simulink model "sl_groundvehicleDynamics"  (R2025a)
settings: Solver=ode45  StartTime=0.0  StopTime=2000  RelTol=1e-5  EnableMultiTasking=on
InitFcn:
  | mdl_robot;
values from neighbouring files (symbols this model uses):
  Ordered_Waypoints = cell2mat({WP_List.Pos}')    [Waypoint_Generator.m]
undefined symbols (not defined in the file or in its folder): DiscIntNeverNeededParam, robot
libraries: simulink x4, mobileRoboticsLib x3, simulink_extras x2
settings Model: Creator=sriramn  LastModifiedBy=Education Account
settings SolverCC: ZeroCrossAlgorithm=Adaptive  AlgebraicLoopSolver=TrustRegion
settings DataIOCC: LimitDataPoints=on  SaveFormat=Array  ReturnWorkspaceOutputs=off
settings OptimizationCC: ReuseModelBlockBuffer=off  LifeSpan=inf
settings DebuggingCC: SolverPrmCheckMsg=warning  UnconnectedInputMsg=warning  UnconnectedOutputMsg=warning  UnconnectedLineMsg=warning  AllowSymbolicDim=off  SFUnexpectedBacktrackingDiag=warning  SFNoUnconditionalDefaultTransitionDiag=warning  SFExecutionAtInitializationDiag=none  UnderSpecifiedDimensionMsg=warning  ArithmeticOperatorsInVariantConditions=warning
settings HardwareCC: ProdBitPerPointer=32.0  ProdBitPerSizeT=32.0  ProdBitPerPtrDiffT=32.0  ProdLargestAtomicFloat=None  ProdIntDivRoundTo=Undefined  ProdEndianess=Unspecified  ProdWordSize=32.0  ProdHWDeviceType=32-bit Generic
settings ModelReferenceCC: EnableRefExpFcnMdlSchedulingChecks=on  ModelReferenceMinAlgLoopOccurrences=on  PropagateSignalLabelsOutOfModel=off
settings SFSimCC: SimUseLocalCustomCode=off  CustomCodeUndefinedFunction=UseInterfaceOnly
settings RTWCC: RTWUseLocalCustomCode=off  GPUComputeCapability=3.5
settings CodeAppCC: StateflowObjectComments=on
settings GRTTargetCC: TargetLangStandard=C89/C90 (ANSI)
settings ConfigComp: CovMetricSettings=dw  CovSaveCumulativeToWorkspaceVar=on  CovSaveSingleToWorkspaceVar=on  CovExternalEMLEnable=off  CovSFcnEnable=off
settings SimscapeCC: SimscapeNormalizeSystem=off
settings ConfigurationSet: Description=SimMechanics 2G
settings ExplorerConfigSet: InternalSimMechanicsExplorerSettings="<ExplorerConfiguration><canonicalview>planar_xy</canonicalview><AnimationSetting><BasePlaybackSpeed>1.0</BasePlaybackSpeed><PlaybackSpeedFactor>1.0</PlaybackSpeedFactor></AnimationSetting><TilePanel><TileInfo><Tiles Columns=\"1\" Count=\"1\" Rows=\"1\"><Column Left=\"2\" Weight=\"1\"/><Column Left=\"1628\"/><Row Top=\"2\" Weight=\"1\"/><Row Top=\"1072\"/><Tile Height=\"1\" Width=\"1\" X=\"0\" Y=\"0\"/></Tiles></TileInfo><SceneInfo><SceneViewer><BGColor><R>0.60000002384185791</R><G>0.60000002384185791</G><B>0.60000002384185791</B></BGColor><Camera><Position><X>0.22951840878551699</X><Y>0.32651610611526627</Y><Z>-0.27215421354393321</Z></Position><Center><X>-0.15775714411666431</X><Y>-0.15462825985839526</Y><Z>0.065702552916005602</Z></Center><Up><X>-0.56030137557930915</X><Y>0.72817587161684794</Y><Z>0.39474329445726858</Z></Up><Left>-0.21481383955700509</Left><Right>0.21481383955700509</Right><Bottom>-0.27569784609469139</Bottom><Top>0.27569784609469139</Top></Camera></SceneViewer></SceneInfo></TilePanel></ExplorerConfiguration>"

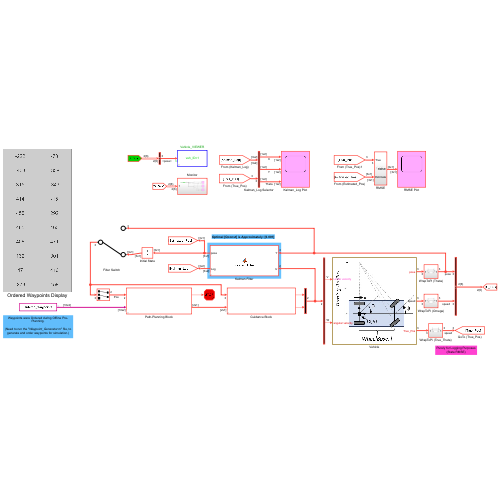
[thumbnail: Simulink's stored preview of the top-level diagram]
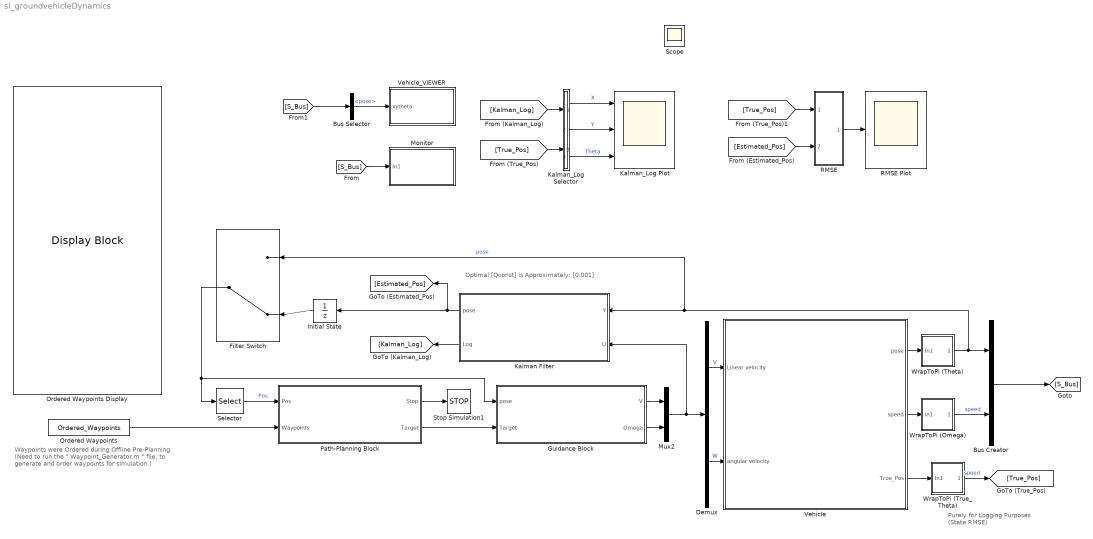
== system sl_groundvehicleDynamics ==
  note: Optimal [Qconst] is Approximately: [0.001]
  note: Waypoints were Ordered during Offline Pre-Planning.
      |
      | (Need to run the " Waypoint_Generator.m " file, to generate and order waypoints for simulation.)
  note: Purely for Logging Purposes
      | (State RMSE)
  Bus Creator : BusCreator  Inputs=2
  Bus Selector : BusSelector  OutputSignals=pose
  Demux : Demux  Outputs=2
  Filter Switch : ManualSwitch  CurrentSetting=0
  Guidance Block : MATLAB Function  TreatAsAtomicUnit=on  mask{Vc=10, MaxOmega=90, Kp=10, Kd=0, N=4, dT=0.05}
      mask prompts: Vc "Linear Velocity (m/s):"; MaxOmega "Maximum Angular Velocity (deg/s):"; Kp "Proportional Gain [Kp]:"; Kd "Derivative Gain [Kd] (ignore):"; N "Navigation Gain [N] (ignore):"; dT "Sample Time [dT]:"
  Initial State : UnitDelay  InitialCondition=[0; 0; 0]  SampleTime=0.05  HasFrameUpgradeWarning=on
  Kalman Filter : MATLAB Function  TreatAsAtomicUnit=on  SystemSampleTime=0.05  mask{sig2_V=10^-3, sig2_W=10^-3, P0_pos=100, P0_theta=100, dT=0.05}
      mask prompts: sig2_V "Linear Velocity Variance [sig2_V]:"; sig2_W "Angular Velocity Variance [sig2_W]:"; P0_pos "Initial Position Variance [P0_pos]:"; P0_theta "Initial Heading Variance [P0_theta]:"; dT "Sample Time [dT]:"
  Kalman_Log Plot : Scope  NumInputPorts=3
      settings: SampleTime=0.05  TimeSpan=350  ActiveDisplayYMinimum=-0.45488119893113321  ActiveDisplayYMaximum=0.48875254754884168
  Kalman_Log Selector : Subsystem
  Monitor : Subsystem
  Mux2 : Mux  Inputs=2
  Ordered Waypoints : Constant  Value=Ordered_Waypoints  VectorParams1D=off
  Ordered Waypoints Display : DisplayBlock  LabelPosition=Hide  Transparency=1  GridColor=[0.502, 0.502, 0.502]
  Path-Planning Block : MATLAB Function  TreatAsAtomicUnit=on  mask{LookAhead=5, WP_Thresh=20}
      mask prompts: LookAhead "Look-Ahead Distance [Ahead]:"; WP_Thresh "WayPoint Threshold [WP_Thresh]:"
  RMSE : Subsystem
  RMSE Plot : Scope
      settings: SampleTime=0.05  TimeSpan=700  Title=State Estimation RMSE  ActiveDisplayYMinimum=-0.13363764478764484  ActiveDisplayYMaximum=1.9663623552123544  YLabel=RMSE  DataLoggingVariableName=ScopeData3
  Selector : Selector  InputPortWidth=3  IndexOptions=Index vector (dialog)  Indices=[1 2]  OutputSizes=1
  Stop Simulation1 : Stop
  Vehicle : Subsystem
      mask Display: image('vehicle.jpg');
  Vehicle_VIEWER : Subsystem  mask{wp_mat=[-500, 500; -500, 500]', veh_ID_num=1, veh_init_xytheta=[robot.X robot.Y robot.Theta], Ts=0.5}
      mask prompts: wp_mat "Waypoint matrix for arena [x_col, y_col] (m)"; veh_ID_num "Vehicle ID number"; veh_init_xytheta "Initial pose [x,y,theta]"; Ts "Sample time for updating animation (secs)"
      mask TypeOptions veh_ID_num: 1 | 2 | 3 | 4
      mask DialogControl Control2 Prompt: Animate simulation of Differential Drive Robot (DDR)
      mask Display: fprintf('veh_ID=%d',veh_ID_num);
  WrapToPi (Omega) : Subsystem
  WrapToPi (Theta) : Subsystem
  WrapToPi (True_Theta) : Subsystem
  Scope : Scope
      settings: ActiveDisplayYMinimum=0.07  ActiveDisplayYMaximum=0.09
  wires:
  [S_Bus] -> Monitor/1(In1)
  [S_Bus] -> Bus Selector/1
  Vehicle/2(speed) -> WrapToPi (Omega)/1(In1)
  Bus Creator/1 -> [S_Bus]
  Bus Selector/1 -> Vehicle_VIEWER/1(xytheta)  "<pose>"
  Demux/1 -> Vehicle/1(Linear velocity)  "V"
  Guidance Block/2(Omega) -> Mux2/2
  Guidance Block/1(V) -> Mux2/1
  Demux/2 -> Vehicle/2(angular velocity)  "W"
  Mux2/1 -> Kalman Filter/2(U), Demux/1
  Path-Planning Block/2(Target) -> Guidance Block/2(Target)
  Ordered Waypoints/1 -> Path-Planning Block/2(Waypoints)
  Vehicle/1(pose) -> WrapToPi (Theta)/1(In1)
  Path-Planning Block/1(Stop) -> Stop Simulation1/1
  Kalman Filter/1(pose) -> [Estimated_Pos], Initial State/1
  Filter Switch/1 -> Guidance Block/1(pose), Selector/1
  Selector/1 -> Path-Planning Block/1(Pos)  "Pos"
  Kalman_Log Selector/2(Y) -> Kalman_Log Plot/2  "Y"
  Kalman_Log Selector/1(X) -> Kalman_Log Plot/1  "X"
  Kalman_Log Selector/3(Theta) -> Kalman_Log Plot/3  "Theta"
  [Kalman_Log] -> Kalman_Log Selector/1(Log)
  WrapToPi (Theta)/1(Out1) -> Bus Creator/1, Kalman Filter/1(Y), Filter Switch/1  "pose"
  WrapToPi (Omega)/1(Out1) -> Bus Creator/2  "speed"
  Initial State/1 -> Filter Switch/2
  Kalman Filter/2(Log) -> [Kalman_Log]
  Vehicle/3(True_Pos) -> WrapToPi (True_Theta)/1(In1)
  [True_Pos] -> Kalman_Log Selector/2(True_Pos)
  WrapToPi (True_Theta)/1(Out1) -> [True_Pos]  "speed"
  [True_Pos] -> RMSE/1(True)
  [Estimated_Pos] -> RMSE/2(Estimate)
  RMSE/1(RMSE) -> RMSE Plot/1

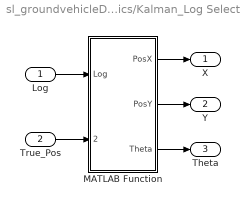
== system sl_groundvehicleDynamics/Kalman_Log Selector ==
  Log : Inport
  True_Pos : Inport  Port=2
  MATLAB Function : MATLAB Function  TreatAsAtomicUnit=on
  X : Outport
  Y : Outport  Port=2
  Theta : Outport  Port=3
  wires:
  MATLAB Function/1(PosX) -> X/1
  MATLAB Function/2(PosY) -> Y/1
  MATLAB Function/3(Theta) -> Theta/1
  Log/1 -> MATLAB Function/1(Log)
  True_Pos/1 -> MATLAB Function/2(True_Pos)

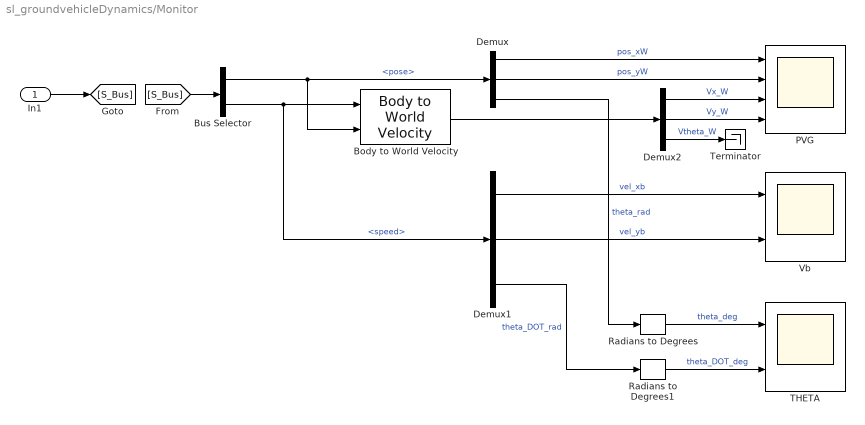
== system sl_groundvehicleDynamics/Monitor ==
  In1 : Inport
  Body to World Velocity : mobileRoboticsLib/Utilities/Body to World Velocity
      settings: SourceProductName=Mobile Robotics Simulation Toolbox
  Bus Selector : BusSelector  OutputSignals=pose,speed
  Demux : Demux  Outputs=3
  Demux1 : Demux  Outputs=3
  Demux2 : Demux  Outputs=3
  PVG : Scope  NumInputPorts=4
      settings: ActiveDisplayYMinimum=-5.1706239874781605  ActiveDisplayYMaximum=31.754450302209349
  Radians to Degrees : simulink_extras/Transformations/Radians to Degrees
  Radians to Degrees1 : simulink_extras/Transformations/Radians to Degrees
  THETA : Scope  NumInputPorts=2
      settings: ActiveDisplayYMinimum=-8.72937  ActiveDisplayYMaximum=60.06611  DataLoggingVariableName=ScopeData2
  Terminator : Terminator
  Vb : Scope  NumInputPorts=2
      settings: ActiveDisplayYMinimum=0.05577  ActiveDisplayYMaximum=0.8929
  wires:
  In1/1 -> [S_Bus]
  [S_Bus] -> Bus Selector/1
  Demux/1 -> PVG/1  "pos_xW"
  Demux/2 -> PVG/2  "pos_yW"
  Radians to Degrees1/1 -> THETA/2  "theta_DOT_deg"
  Radians to Degrees/1 -> THETA/1  "theta_deg"
  Demux1/3 -> Radians to Degrees1/1  "theta_DOT_rad"
  Demux/3 -> Radians to Degrees/1  "theta_rad"
  Bus Selector/1 -> Body to World Velocity/2, Demux/1  "<pose>"
  Bus Selector/2 -> Demux1/1, Body to World Velocity/1  "<speed>"
  Body to World Velocity/1 -> Demux2/1
  Demux2/1 -> PVG/3  "Vx_W"
  Demux2/2 -> PVG/4  "Vy_W"
  Demux1/1 -> Vb/1  "vel_xb"
  Demux1/2 -> Vb/2  "vel_yb"
  Demux2/3 -> Terminator/1  "Vtheta_W"

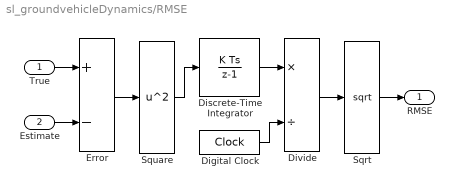
== system sl_groundvehicleDynamics/RMSE ==
  True : Inport
  Estimate : Inport  Port=2
  Digital Clock : DigitalClock  SampleTime=0.05
  Discrete-Time Integrator : DiscreteIntegrator  SampleTime=0.05  ICPrevOutput=DiscIntNeverNeededParam  ICPrevScaledInput=DiscIntNeverNeededParam
  Divide : Product  Inputs=*/
  Error : Sum  Inputs=+-
  Sqrt : Sqrt
  Square : Math  Operator=square
  RMSE : Outport
  wires:
  True/1 -> Error/1
  Estimate/1 -> Error/2
  Divide/1 -> Sqrt/1
  Digital Clock/1 -> Divide/2
  Square/1 -> Discrete-Time Integrator/1
  Error/1 -> Square/1
  Discrete-Time Integrator/1 -> Divide/1
  Sqrt/1 -> RMSE/1

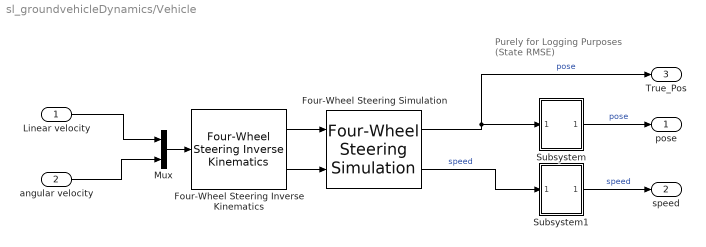
== system sl_groundvehicleDynamics/Vehicle ==
  note: Purely for Logging Purposes
      | (State RMSE)
  Linear velocity : Inport
  angular velocity : Inport  Port=2
  Four-Wheel Steering Inverse Kinematics : mobileRoboticsLib/Kinematic Models/Four-Wheel Steering/Four-Wheel Steering Inverse Kinematics  wheelRadius=0.1  frontWheelDist=0.25  rearWheelDist=0.25  ikMode=Front Steering
      settings: SourceProductName=Mobile Robotics Simulation Toolbox
  Four-Wheel Steering Simulation : mobileRoboticsLib/Kinematic Models/Four-Wheel Steering/Four-Wheel Steering Simulation  wheelRadius=0.1  frontWheelDist=0.25  rearWheelDist=0.25  initX=robot.X  initY=robot.Y  initAngle=robot.Theta  Ts=0.05
      settings: SourceProductName=Mobile Robotics Simulation Toolbox
  Mux : Mux  Inputs=2
  Subsystem : Subsystem
  Subsystem1 : Subsystem
  pose : Outport  VectorParamsAs1DForOutWhenUnconnected=off
  speed : Outport  Port=2
  True_Pos : Outport  Port=3  VectorParamsAs1DForOutWhenUnconnected=off
  wires:
  angular velocity/1 -> Mux/2
  Linear velocity/1 -> Mux/1
  Mux/1 -> Four-Wheel Steering Inverse Kinematics/1
  Four-Wheel Steering Simulation/1 -> True_Pos/1, Subsystem/1(In1)  "pose"
  Four-Wheel Steering Simulation/2 -> Subsystem1/1(In1)  "speed"
  Four-Wheel Steering Inverse Kinematics/1 -> Four-Wheel Steering Simulation/1
  Four-Wheel Steering Inverse Kinematics/2 -> Four-Wheel Steering Simulation/2
  Subsystem/1(pose) -> pose/1  "pose"
  Subsystem1/1(speed) -> speed/1  "speed"

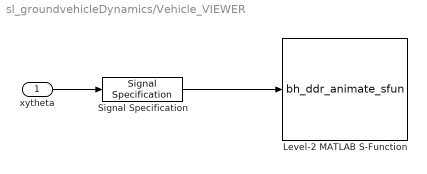
== system sl_groundvehicleDynamics/Vehicle_VIEWER ==
  xytheta : Inport
  Level-2 MATLAB S-Function : M-S-Function  FunctionName=bh_ddr_animate_sfun  Parameters=Ts, Ordered_Waypoints, veh_ID_num, veh_init_xytheta
  Signal Specification : SignalSpecification  Dimensions=3
  wires:
  xytheta/1 -> Signal Specification/1
  Signal Specification/1 -> Level-2 MATLAB S-Function/1

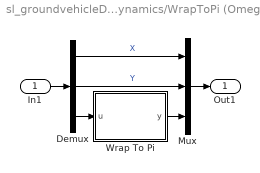
== system sl_groundvehicleDynamics/WrapToPi (Omega) ==
  In1 : Inport
  Demux : Demux  Outputs=3
  Mux : Mux  Inputs=3
  Wrap To Pi : MATLAB Function  TreatAsAtomicUnit=on
  Out1 : Outport
  wires:
  In1/1 -> Demux/1
  Mux/1 -> Out1/1
  Demux/1 -> Mux/1  "X"
  Demux/2 -> Mux/2  "Y"
  Demux/3 -> Wrap To Pi/1(u)
  Wrap To Pi/1(y) -> Mux/3

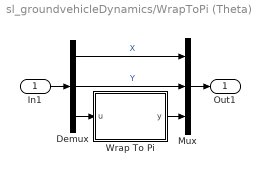
== system sl_groundvehicleDynamics/WrapToPi (Theta) ==
  In1 : Inport
  Demux : Demux  Outputs=3
  Mux : Mux  Inputs=3
  Wrap To Pi : MATLAB Function  TreatAsAtomicUnit=on
  Out1 : Outport
  wires:
  In1/1 -> Demux/1
  Mux/1 -> Out1/1
  Demux/1 -> Mux/1  "X"
  Demux/2 -> Mux/2  "Y"
  Demux/3 -> Wrap To Pi/1(u)
  Wrap To Pi/1(y) -> Mux/3

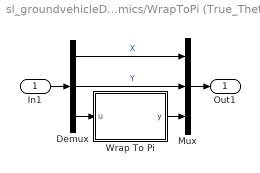
== system sl_groundvehicleDynamics/WrapToPi (True_Theta) ==
  In1 : Inport
  Demux : Demux  Outputs=3
  Mux : Mux  Inputs=3
  Wrap To Pi : MATLAB Function  TreatAsAtomicUnit=on
  Out1 : Outport
  wires:
  Wrap To Pi/1(y) -> Mux/3
  Demux/3 -> Wrap To Pi/1(u)
  Demux/2 -> Mux/2  "Y"
  Demux/1 -> Mux/1  "X"
  Mux/1 -> Out1/1
  In1/1 -> Demux/1

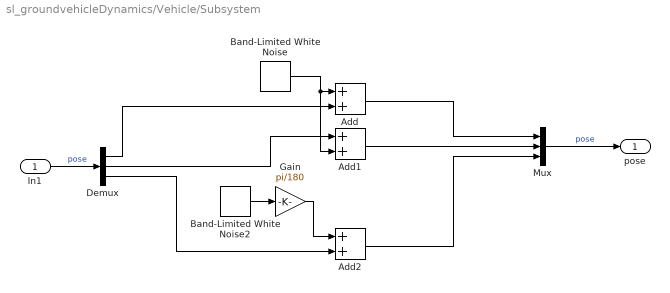
== system sl_groundvehicleDynamics/Vehicle/Subsystem ==
  In1 : Inport
  Add : Sum
  Add1 : Sum
  Add2 : Sum
  Band-Limited White Noise : simulink/Sources/Band-Limited White Noise  Cov=[0.001]  Ts=0.1  seed=[23341]
  Band-Limited White Noise2 : simulink/Sources/Band-Limited White Noise  Cov=[0.41]  Ts=0.1  seed=[23341]
  Demux : Demux  Outputs=3
  Gain : Gain  Gain=pi/180
  Mux : Mux  Inputs=3
  pose : Outport
  wires:
  Add1/1 -> Mux/2
  Add2/1 -> Mux/3
  Demux/2 -> Add1/1
  Band-Limited White Noise2/1 -> Gain/1
  Demux/3 -> Add2/2
  Band-Limited White Noise/1 -> Add1/2, Add/1
  In1/1 -> Demux/1  "pose"
  Demux/1 -> Add/2
  Gain/1 -> Add2/1
  Mux/1 -> pose/1  "pose"
  Add/1 -> Mux/1

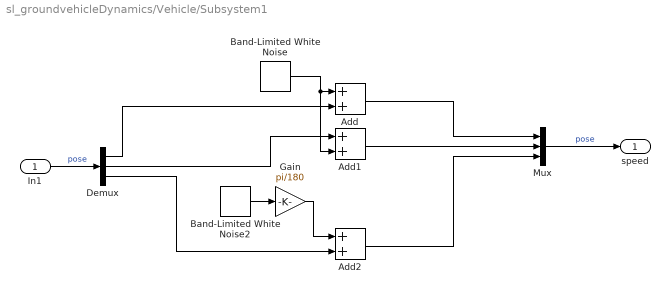
== system sl_groundvehicleDynamics/Vehicle/Subsystem1 ==
  In1 : Inport
  Add : Sum
  Add1 : Sum
  Add2 : Sum
  Band-Limited White Noise : simulink/Sources/Band-Limited White Noise  Cov=[0.001]  Ts=0.1  seed=[23341]
  Band-Limited White Noise2 : simulink/Sources/Band-Limited White Noise  Cov=[0.41]  Ts=0.1  seed=[23341]
  Demux : Demux  Outputs=3
  Gain : Gain  Gain=pi/180
  Mux : Mux  Inputs=3
  speed : Outport
  wires:
  Add1/1 -> Mux/2
  Add2/1 -> Mux/3
  Demux/2 -> Add1/1
  Band-Limited White Noise2/1 -> Gain/1
  Demux/3 -> Add2/2
  Band-Limited White Noise/1 -> Add1/2, Add/1
  In1/1 -> Demux/1  "pose"
  Demux/1 -> Add/2
  Gain/1 -> Add2/1
  Mux/1 -> speed/1  "pose"
  Add/1 -> Mux/1

== matlab function sl_groundvehicleDynamics/Path-Planning Block ==
  data: Stop output; Target output; Pos input; Waypoints input; WP_Thresh parameter; LookAhead parameter
function [Stop, Target] = Path_Planning(Pos, Waypoints, WP_Thresh, LookAhead)


persistent WP_List;
persistent N_WPs;
persistent Target_WP_Idx;


Stop = 0;

% % X-Y Position of the Robot:
% Pos = [pose(1), pose(2)];


%% Parsing and Initialisation of Waypoints:

if isempty(WP_List)

    N_WPs = size(Waypoints, 1);

    WP_List = repmat(struct("Pos", zeros(2, 1), "Visited", false, "Vect", zeros(2, 1), "Len", 0, "Dir", zeros(2, 1)), 1, N_WPs);

    % Turning the List of WPs into a Struct Array:
    for k = 1:N_WPs

        WP_List(k).Pos = Waypoints(k, :).';

        if k ~= 1,  WP_List(k).Vect = Waypoints(k, :).' - Waypoints(k-1, :).';
        else,       WP_List(k).Vect = Waypoints(k, :).' - Pos;              % [Pos] here is the Initial Pos of the Robot.
        end

        WP_List(k).Len = norm(WP_List(k).Vect);
        WP_List(k).Dir = WP_List(k).Vect / WP_List(k).Len;
    
    end

    Target_WP_Idx = 1;
end


%% Indexing Target WP:

if sqrt( (WP_List(Target_WP_Idx).Pos(1)-Pos(1))^2 + (WP_List(Target_WP_Idx).Pos(2)-Pos(2))^2 ) < WP_Thresh

    WP_List(Target_WP_Idx).Visited = true;

    if (Target_WP_Idx == N_WPs), Stop = 1;
    else, Target_WP_Idx = Target_WP_Idx + 1;
    end

end


%% Calculating Vector Projection onto Segment + LookAhead:


Dot_Product_Proj =  dot(WP_List(Target_WP_Idx).Dir, (Pos - WP_List(Target_WP_Idx).Pos));

Target = WP_List(Target_WP_Idx).Pos + (min((Dot_Product_Proj + LookAhead), WP_List(Target_WP_Idx).Len) * WP_List(Target_WP_Idx).Dir);

== matlab function sl_groundvehicleDynamics/Kalman Filter ==
  data: Y input; U input size=2; P0_pos parameter; P0_theta parameter; pose output; sig2_V parameter; sig2_W parameter; dT parameter; Log output
function [pose, Log] = Kalman_Filter(Y, U, P0_pos, P0_theta, sig2_V, sig2_W, dT)

%{

Measurement     [Y]     =   [Xpos; Ypos; Theta]
Command Output  [U]     =   [V; W]

%}


%% %%%%%%%%%%%%%%%%%%%%%%%%%%%%%%%%%%%%%%%%%%%%%%%%%%%%%%%%%%%%%%%%%%%%%%%%
%% Configs:

persistent Xh P
persistent R Q
persistent G
if isempty(Xh)

    % Model State [Xh]:
    Xh   = zeros(3, 1);

    % Model Co-Variance [P]:
    P   = diag([P0_pos, P0_pos, P0_theta]);

    % Known Variances:
    sig2_Xpos   = 0.1;          % Xpos R-Var.
    sig2_Ypos   = 0.1;          % Ypos R-Var.
    sig2_Theta  = deg2rad(2);   % Theta R-Var.

    % Measurement Noise Variance [R]:
    R   = diag([sig2_Xpos, sig2_Ypos, sig2_Theta]);     % Measurement Variance (R-Var).
    
    % Process Noise Variance [Q]:
    Q   = diag([sig2_V, sig2_V, sig2_W]);               % Command Variance (Q-Var).
    


    % State Transition Matrix [F]:
    % F   = eye(3);

    % Input Distribution Matrix [G]:
    G   = dT * eye(3);

    % Output Matrix [C]:
    % C   = eye(3);

    % Output Matrix [D]:
    % D   = 0;

end


%% %%%%%%%%%%%%%%%%%%%%%%%%%%%%%%%%%%%%%%%%%%%%%%%%%%%%%%%%%%%%%%%%%%%%%%%%
%% Prediction [k|k-1]:


% Command Input [U] (2x1)->(3x1):
InputExpansion  = [ cos(Xh(3)),     0;
                    sin(Xh(3)),     0;
                    0,              1  ];

U = InputExpansion * U;


% State Prediction [Xh_]:
Xh_ = Xh + G*U;

% Co-Variance Prediction [P_]:
P_ = P + Q;

% Measurement Prediction [Y_]:
Y_ = Xh_;


%% Measurement [k|k]:

% Innovation: (Measurement Error)
Innov       = Y - Y_;
Innov(3)    = wrapToPi(Innov(3));      % Wrap Theta Error to [-pi, pi] to avoid jumps.

% Kalman Gain [K]:
K = P_ / (P_ + R);

% State Estimation [Xh]:
Xh       = Xh_ + K*(Innov);
Xh(3)    = wrapToPi(Xh(3));

% Co-Variance Estimation [P]:
P = (eye(3) - K)*P_;


%% %%%%%%%%%%%%%%%%%%%%%%%%%%%%%%%%%%%%%%%%%%%%%%%%%%%%%%%%%%%%%%%%%%%%%%%%
%% Output:

pose = Xh;   % Column Vector [3x1]


%% Logging:

% Log = diag(K);

Log = [Y, Xh];



%% %%%%%%%%%%%%%%%%%%%%%%%%%%%%%%%%%%%%%%%%%%%%%%%%%%%%%%%%%%%%%%%%%%%%%%%%
end

== matlab function sl_groundvehicleDynamics/WrapToPi (Theta)/Wrap To Pi ==
  data: u input; y output
function y = WrapToPi(u)

y = wrapToPi(u);

== matlab function sl_groundvehicleDynamics/Guidance Block ==
  data: V output; pose input; Omega output; Target input; Vc parameter; Kp parameter; Kd parameter; N parameter; MaxOmega parameter; dT parameter
function [V, Omega] = Guidance(pose, Target, Vc, Kp, Kd, N, MaxOmega, dT)

persistent Last_Delta;
persistent Last_RTP;


%% Velocity:

% Linear Constant Velocity [V]:
V = Vc;


%% Range and Heading:

% Flight Path Angle [Gamma], (rad):
Gamma = pose(3);


% Relative Target Position [RTP] in the inertial frame, (m):
RTP = [(Target(1) - pose(1));... % dx
    (Target(2) - pose(2))];      % dy

% Range to Target [Range], (m):
Range = norm(RTP);

% Line-Of-Sight [Lambda] Angle, (rad):
Lambda = atan2(RTP(2),RTP(1));


%% Proportional [P] (Pure Pursuite):

% Heading Error [Delta], (rad):
Delta = Lambda - Gamma;
if      (Delta < -pi),  Delta = Delta + 2*pi;
elseif  (Delta > +pi),  Delta = Delta - 2*pi;
end


%% Derivitive [D] (Proportional Navigation):

if isempty(Last_Delta), Last_Delta  = Delta;   end
if isempty(Last_RTP),   Last_RTP    = RTP;     end

Delta_dot   = (Delta - Last_Delta) ./ dT;                                   % Delta_dot     - Heading Error Time Derivitive.
RTP_dot     = (RTP - Last_RTP) ./ dT;                                       % RTP_dot       - Relative Target Position Time Derivitive.
Range_dot   = norm(RTP_dot);                                                % Range_dot     - Distance to Target Time Derivitive
Lambda_dot  = ( (RTP(1)*RTP_dot(2)) - (RTP(2)*RTP_dot(1)) ) / ( Range^2 );  % Lambda_dot    - LOS Angle Time Derivitive.

Last_Delta = Delta;
Last_RTP = RTP;



%% Controller Types:

% if (abs(Delta) > pi/3)
%     Omega = (Kp * Delta) + (Kd * Delta_dot);                                % [PD] Controller (Pure Pursuit).
% else
%     Omega = (N * Lambda_dot);                                               % [D] Controller (Proportional Navigation).
% end



%% Pure Pursuit:

Omega = (Kp * Delta) + (Kd * Delta_dot);                                    % [PD] Controller (Pure Pursuit).


%% Output:

% Clamping Angular-Velocity within a Maximum Magnitude: 
MaxOmega = deg2rad(abs(MaxOmega));
Omega = min(max(Omega, -MaxOmega), MaxOmega);


end

== matlab function sl_groundvehicleDynamics/WrapToPi (Omega)/Wrap To Pi ==
  data: u input; y output
function y = WrapToPi(u)

y = wrapToPi(u);

== matlab function sl_groundvehicleDynamics/WrapToPi (True_Theta)/Wrap To Pi ==
  data: u input; y output
function y = WrapToPi(u)

y = wrapToPi(u);

== matlab function sl_groundvehicleDynamics/Kalman_Log Selector/MATLAB Function ==
  data: Log input; PosX output; True_Pos input; PosY output; Theta output
function [PosX, PosY, Theta] = State_Error(Log, True_Pos)

Xh  = Log(:, 1) - True_Pos;
Y   = Log(:, 2) - True_Pos;


PosX    = [Xh(1), Y(1)];
PosY    = [Xh(2), Y(2)];
Theta   = [Xh(3), Y(3)];
